simulink model "Dynamic_Control"  (R2017b)
settings: Solver=ode5  StartTime=0.0  StopTime=0.25  FixedStep=0.01  RelTol=1e-3
settings Model: Creator=hoadv  LastModifiedBy=lehuu
settings DataIOCC: ReturnWorkspaceOutputs=on
settings SFSimCC: SimUseLocalCustomCode=on
settings RTWCC: RTWUseLocalCustomCode=on

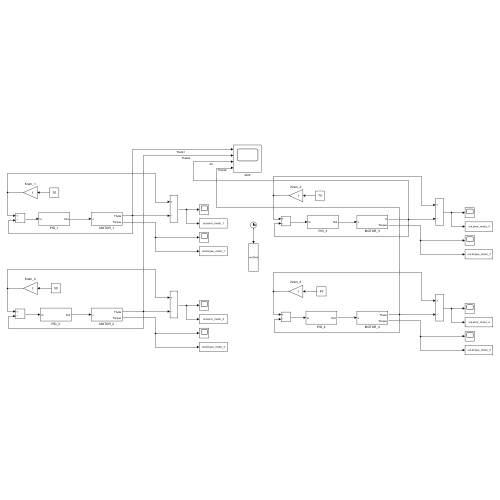
[thumbnail: Simulink's stored preview of the top-level diagram]
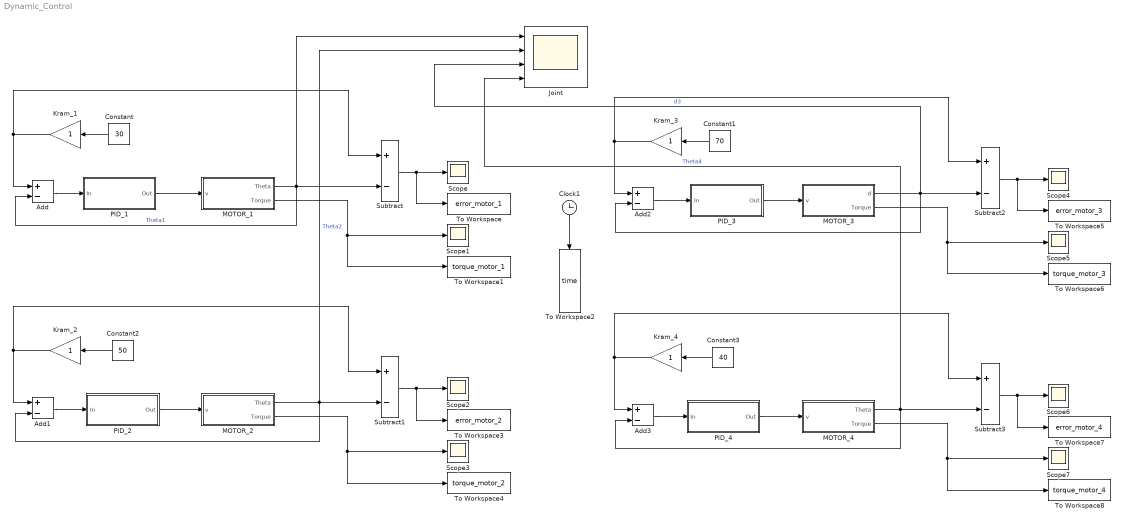
== system Dynamic_Control ==
  Add{,1..3} (4 alike) : Sum  Inputs=+-
  Clock1 : Clock
  Constant : Constant  Value=30
  Constant1 : Constant  Value=70
  Constant2 : Constant  Value=50
  Constant3 : Constant  Value=40
  Joint : Scope  NumInputPorts=4
  Kram_{1..4} (4 alike) : Gain
  MOTOR_1 : Subsystem  mask{L=0.012342, R=3.2645, Jeff=0.01829, Beff=0.019, N=200, Ki=3.8831, Kb=1.1895}
  MOTOR_2 : Subsystem  mask{L=0.012342, R=3.2645, Jeff=0.01829, Beff=0.019, N=100, Ki=3.8831, Kb=1.1895}
  MOTOR_3 : Subsystem  mask{L=0.012342, R=3.2645, Jeff=0.01829, Beff=0.019, N=100, Ki=3.8831, Kb=1.1895}
  MOTOR_4 : Subsystem  mask{L=0.012342, R=3.2645, Jeff=0.01829, Beff=0.019, N=50, Ki=3.8831, Kb=1.1895}
  PID_1 : Subsystem  mask{Kp=10000, Ki=0, Kd=40}
  PID_2 : Subsystem  mask{Kp=5000, Ki=0, Kd=20}
  PID_3 : Subsystem  mask{Kp=3000, Ki=0, Kd=10}
  PID_4 : Subsystem  mask{Kp=3000, Ki=0, Kd=15}
  Scope{,1..7} (8 alike) : Scope
  Subtract{,1..3} (4 alike) : Sum  Inputs=+-
  To Workspace : ToWorkspace  VariableName=error_motor_1  SaveFormat=Timeseries  SampleTime=-1
  To Workspace1 : ToWorkspace  VariableName=torque_motor_1  SaveFormat=Timeseries  SampleTime=-1
  To Workspace2 : ToWorkspace  VariableName=time  SaveFormat=Timeseries  SampleTime=-1
  To Workspace3 : ToWorkspace  VariableName=error_motor_2  SaveFormat=Timeseries  SampleTime=-1
  To Workspace4 : ToWorkspace  VariableName=torque_motor_2  SaveFormat=Timeseries  SampleTime=-1
  To Workspace5 : ToWorkspace  VariableName=error_motor_3  SaveFormat=Timeseries  SampleTime=-1
  To Workspace6 : ToWorkspace  VariableName=torque_motor_3  SaveFormat=Timeseries  SampleTime=-1
  To Workspace7 : ToWorkspace  VariableName=error_motor_4  SaveFormat=Timeseries  SampleTime=-1
  To Workspace8 : ToWorkspace  VariableName=torque_motor_4  SaveFormat=Timeseries  SampleTime=-1
  wires:
  PID_1/1(Out) -> MOTOR_1/1(v)
  Add/1 -> PID_1/1(In)
  MOTOR_1/1(Theta) -> Subtract/2, Add/2, Joint/1  "Theta1"
  Subtract/1 -> To Workspace/1, Scope/1
  Constant/1 -> Kram_1/1
  Kram_1/1 -> Add/1, Subtract/1
  MOTOR_1/2(Torque) -> To Workspace1/1, Scope1/1
  Clock1/1 -> To Workspace2/1
  MOTOR_2/2(Torque) -> To Workspace4/1, Scope3/1
  Kram_2/1 -> Add1/1, Subtract1/1
  Constant2/1 -> Kram_2/1
  MOTOR_2/1(Theta) -> Subtract1/2, Joint/2, Add1/2  "Theta2"
  Subtract1/1 -> To Workspace3/1, Scope2/1
  Add1/1 -> PID_2/1(In)
  PID_2/1(Out) -> MOTOR_2/1(v)
  PID_3/1(Out) -> MOTOR_3/1(v)
  Subtract2/1 -> To Workspace5/1, Scope4/1
  Constant1/1 -> Kram_3/1
  MOTOR_3/1(d) -> Add2/2, Joint/3, Subtract2/2  "d3"
  Kram_3/1 -> Add2/1, Subtract2/1
  Add2/1 -> PID_3/1(In)
  MOTOR_3/2(Torque) -> To Workspace6/1, Scope5/1
  PID_4/1(Out) -> MOTOR_4/1(v)
  Subtract3/1 -> To Workspace7/1, Scope6/1
  Constant3/1 -> Kram_4/1
  MOTOR_4/1(Theta) -> Subtract3/2, Add3/2, Joint/4  "Theta4"
  Kram_4/1 -> Add3/1, Subtract3/1
  Add3/1 -> PID_4/1(In)
  MOTOR_4/2(Torque) -> To Workspace8/1, Scope7/1

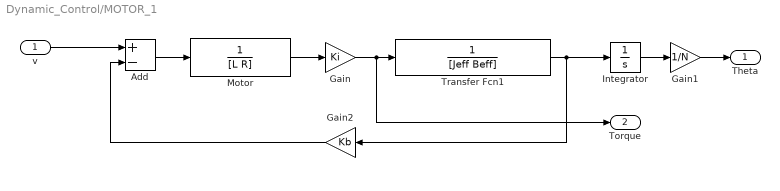
== system Dynamic_Control/MOTOR_1 ==
  v : Inport
  Add : Sum  Inputs=+-
  Gain : Gain  Gain=Ki
  Gain1 : Gain  Gain=1/N
  Gain2 : Gain  Gain=Kb
  Integrator : Integrator
  Motor : TransferFcn  Denominator=[L R]
  Transfer Fcn1 : TransferFcn  Denominator=[Jeff Beff]
  Theta : Outport
  Torque : Outport  Port=2
  wires:
  v/1 -> Add/1
  Add/1 -> Motor/1
  Motor/1 -> Gain/1
  Gain/1 -> Torque/1, Transfer Fcn1/1
  Transfer Fcn1/1 -> Gain2/1, Integrator/1
  Integrator/1 -> Gain1/1
  Gain1/1 -> Theta/1
  Gain2/1 -> Add/2

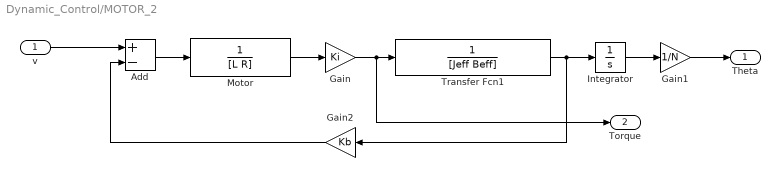
== system Dynamic_Control/MOTOR_2 ==
  v : Inport
  Add : Sum  Inputs=+-
  Gain : Gain  Gain=Ki
  Gain1 : Gain  Gain=1/N
  Gain2 : Gain  Gain=Kb
  Integrator : Integrator
  Motor : TransferFcn  Denominator=[L R]
  Transfer Fcn1 : TransferFcn  Denominator=[Jeff Beff]
  Theta : Outport
  Torque : Outport  Port=2
  wires:
  v/1 -> Add/1
  Add/1 -> Motor/1
  Motor/1 -> Gain/1
  Gain/1 -> Torque/1, Transfer Fcn1/1
  Transfer Fcn1/1 -> Gain2/1, Integrator/1
  Integrator/1 -> Gain1/1
  Gain1/1 -> Theta/1
  Gain2/1 -> Add/2

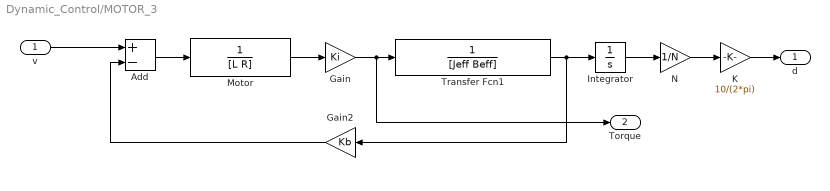
== system Dynamic_Control/MOTOR_3 ==
  v : Inport
  Add : Sum  Inputs=+-
  Gain : Gain  Gain=Ki
  Gain2 : Gain  Gain=Kb
  Integrator : Integrator
  K : Gain  Gain=10/(2*pi)
  Motor : TransferFcn  Denominator=[L R]
  N : Gain  Gain=1/N
  Transfer Fcn1 : TransferFcn  Denominator=[Jeff Beff]
  d : Outport
  Torque : Outport  Port=2
  wires:
  v/1 -> Add/1
  Add/1 -> Motor/1
  Motor/1 -> Gain/1
  Gain/1 -> Torque/1, Transfer Fcn1/1
  Transfer Fcn1/1 -> Gain2/1, Integrator/1
  Integrator/1 -> N/1
  Gain2/1 -> Add/2
  N/1 -> K/1
  K/1 -> d/1

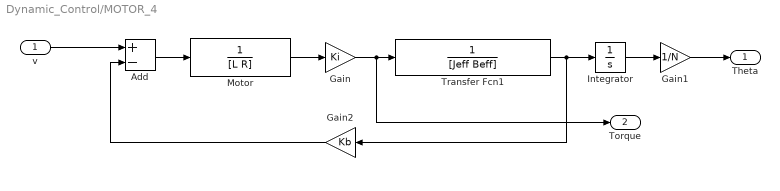
== system Dynamic_Control/MOTOR_4 ==
  v : Inport
  Add : Sum  Inputs=+-
  Gain : Gain  Gain=Ki
  Gain1 : Gain  Gain=1/N
  Gain2 : Gain  Gain=Kb
  Integrator : Integrator
  Motor : TransferFcn  Denominator=[L R]
  Transfer Fcn1 : TransferFcn  Denominator=[Jeff Beff]
  Theta : Outport
  Torque : Outport  Port=2
  wires:
  v/1 -> Add/1
  Add/1 -> Motor/1
  Motor/1 -> Gain/1
  Gain/1 -> Torque/1, Transfer Fcn1/1
  Transfer Fcn1/1 -> Gain2/1, Integrator/1
  Integrator/1 -> Gain1/1
  Gain1/1 -> Theta/1
  Gain2/1 -> Add/2

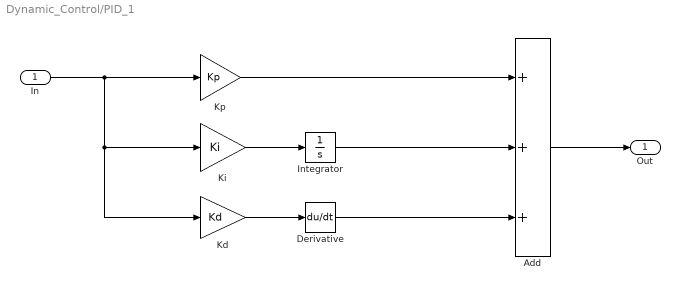
== system Dynamic_Control/PID_1 ==
  In : Inport
  Add : Sum  Inputs=+++
  Derivative : Derivative
  Integrator : Integrator
  Kd : Gain  Gain=Kd
  Ki : Gain  Gain=Ki
  Kp : Gain  Gain=Kp
  Out : Outport
  wires:
  In/1 -> Kd/1, Ki/1, Kp/1
  Add/1 -> Out/1
  Kp/1 -> Add/1
  Ki/1 -> Integrator/1
  Integrator/1 -> Add/2
  Kd/1 -> Derivative/1
  Derivative/1 -> Add/3

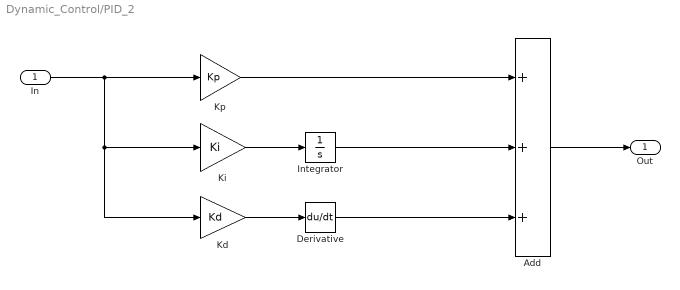
== system Dynamic_Control/PID_2 ==
  In : Inport
  Add : Sum  Inputs=+++
  Derivative : Derivative
  Integrator : Integrator
  Kd : Gain  Gain=Kd
  Ki : Gain  Gain=Ki
  Kp : Gain  Gain=Kp
  Out : Outport
  wires:
  In/1 -> Kd/1, Ki/1, Kp/1
  Add/1 -> Out/1
  Kp/1 -> Add/1
  Ki/1 -> Integrator/1
  Integrator/1 -> Add/2
  Kd/1 -> Derivative/1
  Derivative/1 -> Add/3

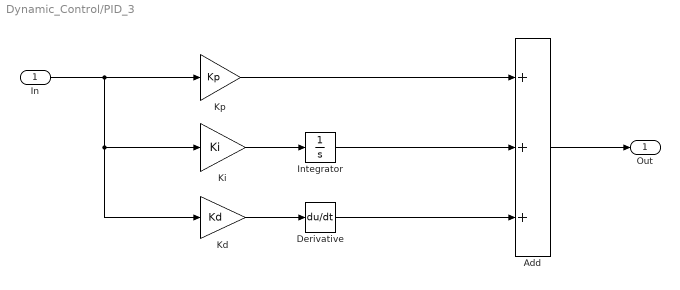
== system Dynamic_Control/PID_3 ==
  In : Inport
  Add : Sum  Inputs=+++
  Derivative : Derivative
  Integrator : Integrator
  Kd : Gain  Gain=Kd
  Ki : Gain  Gain=Ki
  Kp : Gain  Gain=Kp
  Out : Outport
  wires:
  In/1 -> Kd/1, Ki/1, Kp/1
  Add/1 -> Out/1
  Kp/1 -> Add/1
  Ki/1 -> Integrator/1
  Integrator/1 -> Add/2
  Kd/1 -> Derivative/1
  Derivative/1 -> Add/3

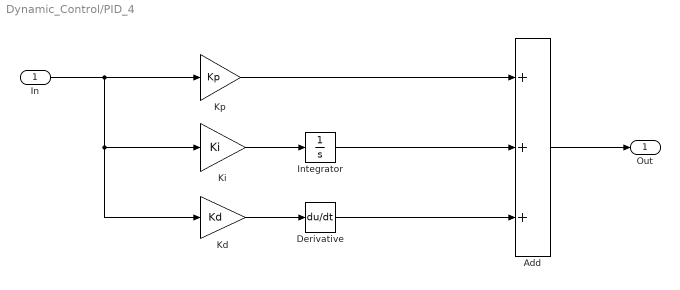
== system Dynamic_Control/PID_4 ==
  In : Inport
  Add : Sum  Inputs=+++
  Derivative : Derivative
  Integrator : Integrator
  Kd : Gain  Gain=Kd
  Ki : Gain  Gain=Ki
  Kp : Gain  Gain=Kp
  Out : Outport
  wires:
  In/1 -> Kd/1, Ki/1, Kp/1
  Add/1 -> Out/1
  Kp/1 -> Add/1
  Ki/1 -> Integrator/1
  Integrator/1 -> Add/2
  Kd/1 -> Derivative/1
  Derivative/1 -> Add/3
